simulink library "carnotUIBK_bus"  (R2023b)
settings: Solver=VariableStepAuto  StartTime=0.0  StopTime=10.0  RelTol=1e-3  EnableMultiTasking=on
values from neighbouring files (symbols this model uses):
  A = 7*10*2    (= 140)    [theta_ground_v1.m]    (also in xlswrite1.m = num2cell(data))
  amb_factor = 1    [DOOR.m]    (also in WALL.m; WINDOW.m = 0)
  area = obj.width * obj.height    [DOOR.m]    (also in RES.m = []; ROOM.m = 0; THERMALZONE.m = area + room(kk).area; WALL.m = area - obj.doors(jj).calc_area())
  B = A/(0.5 * P)    (= 8.23529411765)    [theta_ground_v1.m]
  boundary = BOUNDARY()    [BUILDING.m]    (also in WALL.m = '')
  building = obj    [BUILDING.m]    (also in create_building_automatic.m = building.save(); ini_building_automatic.m = building.add_variant_hvac(building.variant_hvac, hvac); load_building_automatic.m = building.save())
  C = zeros(1,length(d)+1)    [CONSTRUCTION.m]    (also in DOOR.m = [0 0 0]; WALL.m = [0 0 0]; WINDOW.m = [0 0 0])
  control = 2    [GAIN.m]    (also in GAINS.m)
  cp = str2num(value)    [CONSTRUCTION.m]
  height = 0    [DOOR.m]    (also in ROOM.m; THERMALZONE.m; WALL.m; WINDOW.m)
  p = [timevec_weather weather(:,12)]    [BOUNDARY.m]    (also in WEATHER.m = 0; init_carnotUIBK.m = cell2mat(carnotUIBKpaths(i,2)))
  rho = str2num(value)    [CONSTRUCTION.m]    (also in theta_ground_v1.m = 2000)
  type = 1    [CONSTRUCTION.m]    (also in GAINS.m = raw_moisture{ii,3}; STRUCTURE.m = 0)
  view_factor = 1    [DOOR.m]    (also in WINDOW.m = 0)
  wall = []    [ROOM.m]
  z = obj.Z    [WALL.m]    (also in theta_ground_v1.m = 0)
  zone = obj.zone(ind)    [THERMALZONE.m]
undefined symbols (not defined in the file or in its folder): const, Dd, get_building, mdot_air, mdot_CO2, mdot_H2O, mdot_VOC, pos, Qdot_C, Qdot_H, Qdot_I_electricity, Qdot_I_light, Qdot_I_person, Qdot_S, Qdot_T_ground, Qdot_T_internal, Qdot_T_neighbour, Qdot_T_opaque, Qdot_T_window, Qdot_V_infiltration, Qdot_V_mech, Qdot_V_window, Qdotc, Qdotr, r_frame, solar_ratio, solar_ratio1, solar_ratio2, Tc, Tr, Ts, Uvalue, wallsurface, window, window_height, window_heigth, window_width, windowsurface, x_CO2, x_H2O, x_VOC
libraries: $bdroot x134, carnot x87, simulink_extras x14, slpidlib x4, simulink x3
(part 2 of 12)

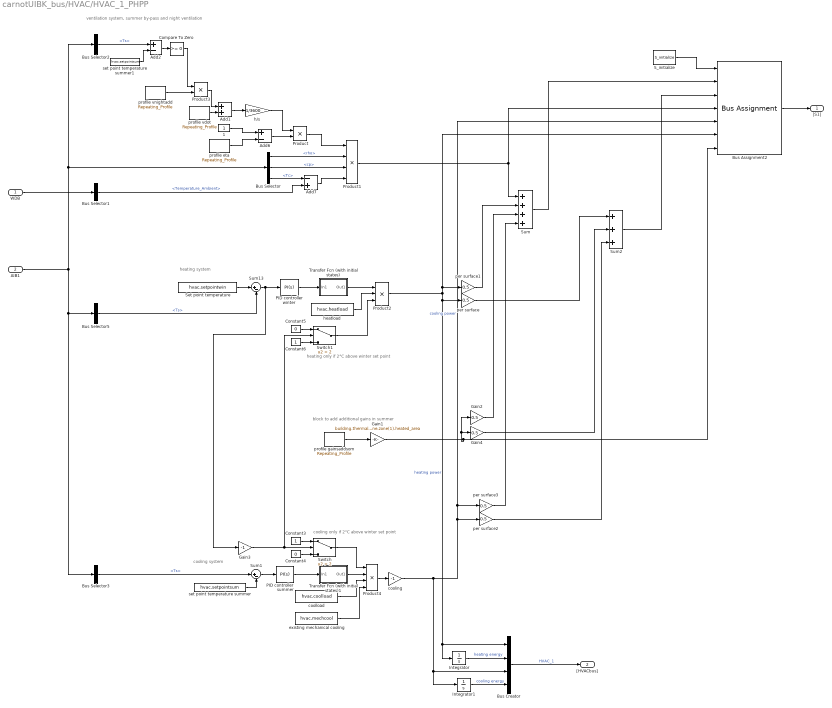
== system carnotUIBK_bus/HVAC/HVAC_1_PHPP ==
  note: cooling only if 2°C above winter set point
  note: block to add additional gains in summer
  note: heating only if 2°C above winter set point
  note: heating system
  note: cooling system
  note: ventilation system, summer by-pass and night ventilation
  WDB : Inport
  AIB1 : Inport  Port=2
  1 : Constant
  Add1 : Sum
  Add2 : Sum  Inputs=+-
  Add6 : Sum  Inputs=+-
  Add7 : Sum  Inputs=-+
  Bus Assignment2 : BusAssignment  AssignedSignals=Qdotc,Qdotr,Qdot_V_mech,Qdot_C,Qdot_H,Qdot_I_person
  Bus Creator : BusCreator  Inputs=4
  Bus Selector : BusSelector  OutputSignals=rho,cp,Tc
  Bus Selector1 : BusSelector  OutputSignals=Temperature_Ambient
  Bus Selector2 : BusSelector  OutputSignals=Ts
  Bus Selector3 : BusSelector  OutputSignals=Ts
  Bus Selector5 : BusSelector  OutputSignals=Ts
  Compare To Zero : simulink/Logic and Bit Operations/Compare To Zero  relop=>=  OutDataTypeStr=boolean
  Constant3 : Constant
  Constant4 : Constant  Value=0
  Constant5 : Constant  Value=0
  Constant6 : Constant
  Gain1 : Gain  Gain=building.thermalzone.zone(1).heated_area  SaturateOnIntegerOverflow=on  OutDataTypeStr=Inherit: Same as input  ParamDataTypeStr=Inherit: Same as input
  Gain2 : Gain  Gain=0.5  SaturateOnIntegerOverflow=on  OutDataTypeStr=Inherit: Same as input  ParamDataTypeStr=Inherit: Same as input
  Gain3 : Gain  Gain=-1  SaturateOnIntegerOverflow=on  OutDataTypeStr=Inherit: Same as input  ParamDataTypeStr=Inherit: Same as input
  Gain4 : Gain  Gain=0.5  SaturateOnIntegerOverflow=on  OutDataTypeStr=Inherit: Same as input  ParamDataTypeStr=Inherit: Same as input
  Integrator : Integrator
  Integrator1 : Integrator
  PID controller summer : slpidlib/PID Controller  Controller=PI  Form=Ideal  TimeDomain=Continuous-time  UseExternalTs=off  SampleTime=-1  IntegratorMethod=Forward Euler  FilterMethod=Forward Euler  ControllerParametersSource=internal  P=hvac.valves.Kp  I=(1/(hvac.valves.Tn*60))  UseKiTs=off  D=0  N=100  UseFilter=on  TunerSelectOption=Transfer Function Based (PID Tuner App)  InitialConditionSource=internal  InitialConditionForIntegrator=0  InitialConditionForFilter=0  DifferentiatorICPrevScaledInput=0  ExternalReset=none  TrackingMode=off  Kt=1  LimitOutput=on  SatLimitsSource=internal  UpperSaturationLimit=hvac.valves.valve_up  LowerSaturationLimit=hvac.valves.valve_low  LinearizeAsGain=off  AntiWindupMode=clamping  Kb=1  LimitIntegrator=off  UpperIntegratorSaturationLimit=inf  LowerIntegratorSaturationLimit=-inf  POutMin=[]  POutMax=[]  IOutMin=[]  IOutMax=[]  DOutMin=[]  DOutMax=[]  NOutMin=[]  NOutMax=[]  SumOutMin=[]  SumOutMax=[]  SaturationOutMin=[]  SaturationOutMax=[]  PParamMin=[]  PParamMax=[]  IParamMin=[]  IParamMax=[]  DParamMin=[]  DParamMax=[]  NParamMin=[]  NParamMax=[]  KbParamMin=[]  KbParamMax=[]  KtParamMin=[]  KtParamMax=[]  KbOutMin=[]  KbOutMax=[]  KtOutMin=[]  KtOutMax=[]  IntegratorOutMin=[]  IntegratorOutMax=[]  FilterOutMin=[]  FilterOutMax=[]  SumI1OutMin=[]  SumI1OutMax=[]  SumI2OutMin=[]  SumI2OutMax=[]  SumI3OutMin=[]  SumI3OutMax=[]  SumI4OutMin=[]  SumI4OutMax=[]  SumDOutMin=[]  SumDOutMax=[]  DifferentiatorOutMin=[]  DifferentiatorOutMax=[]  FilterDiffOutCoefMin=[]  FilterDiffOutCoefMax=[]  ReciprocalOutMin=[]  ReciprocalOutMax=[]  SumDenOutMin=[]  SumDenOutMax=[]  SumNumOutMin=[]  SumNumOutMax=[]  DivideOutMin=[]  DivideOutMax=[]  UdiffTsProdOutMin=[]  UdiffTsProdOutMax=[]  NTsProdOutMin=[]  NTsProdOutMax=[]  UintegralTsProdOutMin=[]  UintegralTsProdOutMax=[]  UngainTsProdOutMin=[]  UngainTsProdOutMax=[]  ClampingZeroOutDataTypeStr=Inherit: Inherit via back propagation  ClampingZeroOutMin=[]  ClampingZeroOutMax=[]  FilterDenConstantOutDataTypeStr=Inherit: Inherit via back propagation  FilterDenConstantOutMin=[]  FilterDenConstantOutMax=[]  PCopyOutDataTypeStr=Inherit: Inherit via back propagation  PCopyOutMin=[]  PCopyOutMax=[]  NCopyOutDataTypeStr=Inherit: Inherit via back propagation  NCopyOutMin=[]  NCopyOutMax=[]  IntegratorContinuousStateAttributes=''  IntegratorStateMustResolveToSignalObject=off  IntegratorRTWStateStorageClass=Auto  FilterContinuousStateAttributes=''  FilterStateMustResolveToSignalObject=off  FilterRTWStateStorageClass=Auto  ParallelPVariant=Passthrough  IdealPVariant=InternalParameters  IVariant=InternalParameters  DVariant=Disabled  IntegratorVariant=Continuous  SatVariant=Enabled  AWVariant=ContClampingIdeal  PCopyVariant=InternalParamsIdeal  TRVariant=Disabled  FdbkBlocksVariant=Forward  IdealPFdbkVariant=Disabled  SatFdbkVariant=Disabled  DerivativeFilterVariant=Disabled  NVariant=Disabled  NCopyVariant=Disabled_SignalSpec  FilterICVariant=Disabled  IntegratorICVariant=InternalICs  ExternalResetVariant=Disabled  TRSumVariant=Passthrough  SumFdbkVariant=Disabled  SumVariant=Sum_PI  TsampFilterVariant=InternalTs  TsampNgainVariant=Passthrough  TsampIntegralVariant=Disabled_SignalSpec  ExternalSaturationOutDataTypeStr=Inherit: Same as second input
  PID controller winter : slpidlib/PID Controller  Controller=PI  Form=Ideal  TimeDomain=Continuous-time  UseExternalTs=off  SampleTime=-1  IntegratorMethod=Forward Euler  FilterMethod=Forward Euler  ControllerParametersSource=internal  P=hvac.valves.Kp  I=(1/(hvac.valves.Tn*60))  UseKiTs=off  D=0  N=100  UseFilter=on  TunerSelectOption=Transfer Function Based (PID Tuner App)  InitialConditionSource=internal  InitialConditionForIntegrator=0  InitialConditionForFilter=0  DifferentiatorICPrevScaledInput=0  ExternalReset=none  TrackingMode=off  Kt=1  LimitOutput=on  SatLimitsSource=internal  UpperSaturationLimit=hvac.valves.valve_up  LowerSaturationLimit=hvac.valves.valve_low  LinearizeAsGain=off  AntiWindupMode=clamping  Kb=1  LimitIntegrator=off  UpperIntegratorSaturationLimit=inf  LowerIntegratorSaturationLimit=-inf  POutMin=[]  POutMax=[]  IOutMin=[]  IOutMax=[]  DOutMin=[]  DOutMax=[]  NOutMin=[]  NOutMax=[]  SumOutMin=[]  SumOutMax=[]  SaturationOutMin=[]  SaturationOutMax=[]  PParamMin=[]  PParamMax=[]  IParamMin=[]  IParamMax=[]  DParamMin=[]  DParamMax=[]  NParamMin=[]  NParamMax=[]  KbParamMin=[]  KbParamMax=[]  KtParamMin=[]  KtParamMax=[]  KbOutMin=[]  KbOutMax=[]  KtOutMin=[]  KtOutMax=[]  IntegratorOutMin=[]  IntegratorOutMax=[]  FilterOutMin=[]  FilterOutMax=[]  SumI1OutMin=[]  SumI1OutMax=[]  SumI2OutMin=[]  SumI2OutMax=[]  SumI3OutMin=[]  SumI3OutMax=[]  SumI4OutMin=[]  SumI4OutMax=[]  SumDOutMin=[]  SumDOutMax=[]  DifferentiatorOutMin=[]  DifferentiatorOutMax=[]  FilterDiffOutCoefMin=[]  FilterDiffOutCoefMax=[]  ReciprocalOutMin=[]  ReciprocalOutMax=[]  SumDenOutMin=[]  SumDenOutMax=[]  SumNumOutMin=[]  SumNumOutMax=[]  DivideOutMin=[]  DivideOutMax=[]  UdiffTsProdOutMin=[]  UdiffTsProdOutMax=[]  NTsProdOutMin=[]  NTsProdOutMax=[]  UintegralTsProdOutMin=[]  UintegralTsProdOutMax=[]  UngainTsProdOutMin=[]  UngainTsProdOutMax=[]  ClampingZeroOutDataTypeStr=Inherit: Inherit via back propagation  ClampingZeroOutMin=[]  ClampingZeroOutMax=[]  FilterDenConstantOutDataTypeStr=Inherit: Inherit via back propagation  FilterDenConstantOutMin=[]  FilterDenConstantOutMax=[]  PCopyOutDataTypeStr=Inherit: Inherit via back propagation  PCopyOutMin=[]  PCopyOutMax=[]  NCopyOutDataTypeStr=Inherit: Inherit via back propagation  NCopyOutMin=[]  NCopyOutMax=[]  IntegratorContinuousStateAttributes=''  IntegratorStateMustResolveToSignalObject=off  IntegratorRTWStateStorageClass=Auto  FilterContinuousStateAttributes=''  FilterStateMustResolveToSignalObject=off  FilterRTWStateStorageClass=Auto  ParallelPVariant=Passthrough  IdealPVariant=InternalParameters  IVariant=InternalParameters  DVariant=Disabled  IntegratorVariant=Continuous  SatVariant=Enabled  AWVariant=ContClampingIdeal  PCopyVariant=InternalParamsIdeal  TRVariant=Disabled  FdbkBlocksVariant=Forward  IdealPFdbkVariant=Disabled  SatFdbkVariant=Disabled  DerivativeFilterVariant=Disabled  NVariant=Disabled  NCopyVariant=Disabled_SignalSpec  FilterICVariant=Disabled  IntegratorICVariant=InternalICs  ExternalResetVariant=Disabled  TRSumVariant=Passthrough  SumFdbkVariant=Disabled  SumVariant=Sum_PI  TsampFilterVariant=InternalTs  TsampNgainVariant=Passthrough  TsampIntegralVariant=Disabled_SignalSpec  ExternalSaturationOutDataTypeStr=Inherit: Same as second input
  Product : Product
  Product1 : Product  Inputs=4
  Product2 : Product  Inputs=3
  Product3 : Product
  Product4 : Product  Inputs=4
  S_initialize : $bdroot/general/S_initialize  SystemSampleTime=-1  VariantActivationTime=update diagram  AllowFlexibleInterface=on  Latency=0  AutoFrameSizeCalculation=off
  Set point temperature : Constant  Value=hvac.setpointwin  VectorParams1D=off
  Sum : Sum  Inputs=++++
  Sum1 : Sum  Inputs=|+-
  Sum13 : Sum  Inputs=|+-
  Sum2 : Sum  Inputs=+++
  Switch : Switch  Criteria=u2 > Threshold  Threshold=2  SaturateOnIntegerOverflow=off  InputSameDT=off
  Switch1 : Switch  Criteria=u2 > Threshold  Threshold=2  SaturateOnIntegerOverflow=off  InputSameDT=off
  Transfer Fcn (with initial states) : Subsystem  mask(Transfer Function with Initial States){N=[1], D=[300  1], X0=0}
      mask prompts: N "Numerator:"; D "Denominator:"; X0 "Initial conditions:"
      mask help: Vector expressions for numerator, and denominator. Coefficients are in descending powers of s.
      mask init:
      | [A,B,C,Dd]=tf2ss(N,D);if (isempty(X0));[m,n]=size(A);X0=zeros(1,m); end;
      mask Help: Specify the initial states for the transfer function.  The state ordering is determined by the m-file tf2ss.  There is no unique mapping of the states in a transfer function to states in a state-space representation.  However, tf2ss will consistently use the same mapping for a given transfer function.
      mask Display: dpoly(N,D,'s')
  Transfer Fcn (with initial states)1 : Subsystem  mask(Transfer Function with Initial States){N=[1], D=[300  1], X0=0}
      mask prompts: N "Numerator:"; D "Denominator:"; X0 "Initial conditions:"
      mask help: Vector expressions for numerator, and denominator. Coefficients are in descending powers of s.
      mask init:
      | [A,B,C,Dd]=tf2ss(N,D);if (isempty(X0));[m,n]=size(A);X0=zeros(1,m); end;
      mask Help: Specify the initial states for the transfer function.  The state ordering is determined by the m-file tf2ss.  There is no unique mapping of the states in a transfer function to states in a state-space representation.  However, tf2ss will consistently use the same mapping for a given transfer function.
      mask Display: dpoly(N,D,'s')
  cooling : Gain  Gain=-1  SaturateOnIntegerOverflow=on  OutDataTypeStr=Inherit: Same as input  ParamDataTypeStr=Inherit: Same as input
  coolload : Constant  Value=hvac.coolload
  existing mechanical cooling : Constant  Value=hvac.mechcool
  h/s : Gain  Gain=1/3600
  heatload : Constant  Value=hvac.heatload
  per surface{,1..3} (4 alike) : Gain  Gain=0.5  SaturateOnIntegerOverflow=on  OutDataTypeStr=Inherit: Same as input  ParamDataTypeStr=Inherit: Same as input
  profile eta : carnot/Load/General/Repeating_Profile  period=hvac.eta.time(end)  rep_seq_t=hvac.eta.time(1:end-1)  rep_seq_d=hvac.eta.duration  rep_seq_y=hvac.eta.value
      settings: SourceProductName=Carnot
  profile gainsaddsom : carnot/Load/General/Repeating_Profile  period=hvac.gainsum.time(end)  rep_seq_t=hvac.gainsum.time(1:end-1)  rep_seq_d=hvac.gainsum.duration  rep_seq_y=hvac.gainsum.value
      settings: SourceProductName=Carnot
  profile vdot : carnot/Load/General/Repeating_Profile  period=hvac.vdot_winsom.time(end)  rep_seq_t=hvac.vdot_winsom.time(1:end-1)  rep_seq_d=hvac.vdot_winsom.duration  rep_seq_y=hvac.vdot_winsom.value
      settings: SourceProductName=Carnot
  profile vnightadd : carnot/Load/General/Repeating_Profile  period=hvac.night_vent_s.time(end)  rep_seq_t=hvac.night_vent_s.time(1:end-1)  rep_seq_d=hvac.night_vent_s.duration  rep_seq_y=hvac.night_vent_s.value
      settings: SourceProductName=Carnot
  set point temperature summer : Constant  Value=hvac.setpointsum  VectorParams1D=off
  set point temperature summer1 : Constant  Value=hvac.setpointsum  VectorParams1D=off
  "[S1]" : Outport  InitialOutput=0  VectorParamsAs1DForOutWhenUnconnected=off
  "[HVACbus]" : Outport  Port=2  InitialOutput=0  VectorParamsAs1DForOutWhenUnconnected=off
  wires:
  profile eta/1 -> Add6/2
  profile vdot/1 -> Add1/2
  1/1 -> Add6/1
  Add6/1 -> Product/2
  Product/1 -> Product1/1
  Bus Selector/1 -> Product1/2  "<rho>"
  Bus Selector/2 -> Product1/3  "<cp>"
  Bus Selector/3 -> Add7/1  "<Tc>"
  Product1/1 -> Sum/1, Bus Assignment2/4
  WDB/1 -> Bus Selector1/1
  Bus Selector1/1 -> Add7/2  "<Temperature_Ambient>"
  Add7/1 -> Product1/4
  h/s/1 -> Product/1
  Sum13/1 -> PID controller winter/1, Gain3/1
  Set point temperature/1 -> Sum13/1
  Bus Selector5/1 -> Sum13/2  "<Ts>"
  PID controller winter/1 -> Transfer Fcn (with initial states)/1(In1)
  heatload/1 -> Product2/2
  per surface/1 -> Sum2/1
  per surface1/1 -> Sum/2
  Transfer Fcn (with initial states)/1(Out1) -> Product2/1
  Add1/1 -> h/s/1
  Product3/1 -> Add1/1
  profile vnightadd/1 -> Product3/2
  Bus Selector2/1 -> Add2/1  "<Ts>"
  set point temperature summer1/1 -> Add2/2
  Add2/1 -> Compare To Zero/1
  Compare To Zero/1 -> Product3/1
  profile gainsaddsom/1 -> Gain1/1
  Gain1/1 -> Gain2/1, Gain4/1, Bus Assignment2/7
  Sum1/1 -> PID controller summer/1
  set point temperature summer/1 -> Sum1/2
  Bus Selector3/1 -> Sum1/1  "<Ts>"
  PID controller summer/1 -> Transfer Fcn (with initial states)1/1(In1)
  coolload/1 -> Product4/3
  Product4/1 -> cooling/1
  per surface2/1 -> Sum2/3
  per surface3/1 -> Sum/4
  Transfer Fcn (with initial states)1/1(Out1) -> Product4/2
  AIB1/1 -> Bus Selector3/1, Bus Selector5/1, Bus Selector/1, Bus Selector2/1
  existing mechanical cooling/1 -> Product4/4
  Constant3/1 -> Switch/1
  Constant4/1 -> Switch/3
  Switch/1 -> Product4/1
  Gain3/1 -> Switch1/2, Switch/2
  Constant5/1 -> Switch1/1
  Constant6/1 -> Switch1/3
  Switch1/1 -> Product2/3
  Bus Creator/1 -> "[HVACbus]"/1  "HVAC_1"
  Integrator/1 -> Bus Creator/2  "heating energy"
  Product2/1 -> Bus Assignment2/6, per surface1/1, Integrator/1, Bus Creator/1, per surface/1  "heating power"
  Integrator1/1 -> Bus Creator/4  "cooling energy"
  cooling/1 -> Bus Creator/3, Integrator1/1, Bus Assignment2/5, per surface3/1, per surface2/1  "cooling power"
  S_initialize/1 -> Bus Assignment2/1
  Gain2/1 -> Sum/3
  Gain4/1 -> Sum2/2
  Sum/1 -> Bus Assignment2/2
  Sum2/1 -> Bus Assignment2/3
  Bus Assignment2/1 -> "[S1]"/1

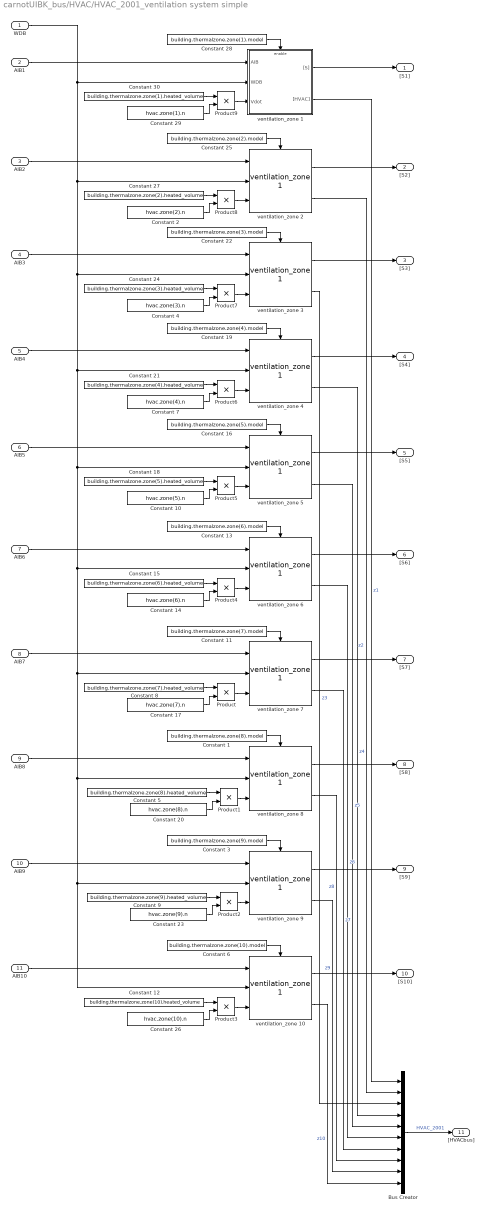
== system carnotUIBK_bus/HVAC/HVAC_2001_ventilation system simple ==
  WDB : Inport
  AIB1 : Inport  Port=2
  AIB2 : Inport  Port=3
  AIB3 : Inport  Port=4
  AIB4 : Inport  Port=5
  AIB5 : Inport  Port=6
  AIB6 : Inport  Port=7
  AIB7 : Inport  Port=8
  "AIB8 " : Inport  Port=9
  AIB9 : Inport  Port=10
  AIB10 : Inport  Port=11
  Bus Creator : BusCreator  Inputs=10
  Constant 1 : Constant  Value=building.thermalzone.zone(8).model  VectorParams1D=off
  Constant 10 : Constant  Value=hvac.zone(5).n  VectorParams1D=off
  Constant 11 : Constant  Value=building.thermalzone.zone(7).model  VectorParams1D=off
  Constant 12 : Constant  Value=building.thermalzone.zone(10).heated_volume  VectorParams1D=off
  Constant 13 : Constant  Value=building.thermalzone.zone(6).model  VectorParams1D=off
  Constant 14 : Constant  Value=hvac.zone(6).n  VectorParams1D=off
  Constant 15 : Constant  Value=building.thermalzone.zone(6).heated_volume  VectorParams1D=off
  Constant 16 : Constant  Value=building.thermalzone.zone(5).model  VectorParams1D=off
  Constant 17 : Constant  Value=hvac.zone(7).n  VectorParams1D=off
  Constant 18 : Constant  Value=building.thermalzone.zone(5).heated_volume  VectorParams1D=off
  Constant 19 : Constant  Value=building.thermalzone.zone(4).model  VectorParams1D=off
  Constant 2 : Constant  Value=hvac.zone(2).n  VectorParams1D=off
  Constant 20 : Constant  Value=hvac.zone(8).n  VectorParams1D=off
  Constant 21 : Constant  Value=building.thermalzone.zone(4).heated_volume  VectorParams1D=off
  Constant 22 : Constant  Value=building.thermalzone.zone(3).model  VectorParams1D=off
  Constant 23 : Constant  Value=hvac.zone(9).n  VectorParams1D=off
  Constant 24 : Constant  Value=building.thermalzone.zone(3).heated_volume  VectorParams1D=off
  Constant 25 : Constant  Value=building.thermalzone.zone(2).model  VectorParams1D=off
  Constant 26 : Constant  Value=hvac.zone(10).n  VectorParams1D=off
  Constant 27 : Constant  Value=building.thermalzone.zone(2).heated_volume  VectorParams1D=off
  Constant 28 : Constant  Value=building.thermalzone.zone(1).model  VectorParams1D=off
  Constant 29 : Constant  Value=hvac.zone(1).n  VectorParams1D=off
  Constant 3 : Constant  Value=building.thermalzone.zone(9).model  VectorParams1D=off
  Constant 30 : Constant  Value=building.thermalzone.zone(1).heated_volume  VectorParams1D=off
  Constant 4 : Constant  Value=hvac.zone(3).n  VectorParams1D=off
  Constant 5 : Constant  Value=building.thermalzone.zone(8).heated_volume  VectorParams1D=off
  Constant 6 : Constant  Value=building.thermalzone.zone(10).model  VectorParams1D=off
  Constant 7 : Constant  Value=hvac.zone(4).n  VectorParams1D=off
  Constant 8 : Constant  Value=building.thermalzone.zone(7).heated_volume  VectorParams1D=off
  Constant 9 : Constant  Value=building.thermalzone.zone(9).heated_volume  VectorParams1D=off
  Product{,1..9} (10 alike) : Product
  ventilation_zone 1 : Subsystem  mask(ACTIVE COMPONENT){co2=400, eta=hvac.zone(1).eta, eta_x=hvac.zone(1).eta_x}
      mask prompts: co2 "CO2 content of air in ppm"; eta "heat recovery efficiency"; eta_x "moisture recovery efficiency"
      mask help:
      | This block represents the AIR VENTILATION from outdoors into a zone.
      |
      | r : rate of nominal air flow between outdoors and indoor, [0,1]
      | [S] : vector for sinks and sources.
      |
      | NOTE: Mass flows of water and CO2 are taken into consideration.
      |
      | ASSUMPTION:
      | Incoming air volume flow is identical to outgoing air volume flow.
      mask init:
      | CO2norm = co2*1e-6;
      mask Help: web(fullfile(path_carnot('help'),'Ventilation_AIV.html'),'-helpbrowser')
      mask Display:
      | plot([0.2 0.35], [0.8 0.7])
      | plot([0.35 0.65], [0.7 0.7])
      | plot([0.65 0.8], [0.7 0.8])
      | plot([0.65 0.8], [0.76 0.8])
      | plot([0.7 0.8], [0.65 0.8])
      | 
      | plot([0.2 0.35], [0.2 0.3])
      | plot([0.35 0.65], [0.3 0.3])
      | plot([0.65 0.8], [0.3 0.2])
      | plot([0.2 0.25], [0.2 0.32])
      | plot([0.2 0.35], [0.2 0.23])
      | 
      | plot ([0.45 0.45], [0 1])
      | plot ([0.55 0.55], [0 1])
      | 
      | plot ([0.45 0.55], [0.2 0.2])
      | plot ([0.45 0.55], [0.8 0.8])
      | 
      | plot ([0.45 0.55], [0 0.2])
      | plot ([0.45 0.55], [0.8 1])
  ventilation_zone 10 : $bdroot/HVAC/HVAC_2001_ventilation system simple/ventilation_zone 1  co2=400  eta=hvac.zone(10).eta  eta_x=hvac.zone(10).eta_x
  ventilation_zone 2 : $bdroot/HVAC/HVAC_2001_ventilation system simple/ventilation_zone 1  co2=400  eta=hvac.zone(2).eta  eta_x=hvac.zone(2).eta_x
  ventilation_zone 3 : $bdroot/HVAC/HVAC_2001_ventilation system simple/ventilation_zone 1  co2=400  eta=hvac.zone(3).eta  eta_x=hvac.zone(3).eta_x
  ventilation_zone 4 : $bdroot/HVAC/HVAC_2001_ventilation system simple/ventilation_zone 1  co2=400  eta=hvac.zone(4).eta  eta_x=hvac.zone(4).eta_x
  ventilation_zone 5 : $bdroot/HVAC/HVAC_2001_ventilation system simple/ventilation_zone 1  co2=400  eta=hvac.zone(5).eta  eta_x=hvac.zone(5).eta_x
  ventilation_zone 6 : $bdroot/HVAC/HVAC_2001_ventilation system simple/ventilation_zone 1  co2=400  eta=hvac.zone(6).eta  eta_x=hvac.zone(6).eta_x
  ventilation_zone 7 : $bdroot/HVAC/HVAC_2001_ventilation system simple/ventilation_zone 1  co2=400  eta=hvac.zone(7).eta  eta_x=hvac.zone(7).eta_x
  ventilation_zone 8 : $bdroot/HVAC/HVAC_2001_ventilation system simple/ventilation_zone 1  co2=400  eta=hvac.zone(8).eta  eta_x=hvac.zone(8).eta_x
  ventilation_zone 9 : $bdroot/HVAC/HVAC_2001_ventilation system simple/ventilation_zone 1  co2=400  eta=hvac.zone(9).eta  eta_x=hvac.zone(9).eta_x
  "[S1]" : Outport  VectorParamsAs1DForOutWhenUnconnected=off
  "[S2]" : Outport  Port=2  VectorParamsAs1DForOutWhenUnconnected=off
  "[S3]" : Outport  Port=3  VectorParamsAs1DForOutWhenUnconnected=off
  "[S4]" : Outport  Port=4  VectorParamsAs1DForOutWhenUnconnected=off
  "[S5]" : Outport  Port=5  VectorParamsAs1DForOutWhenUnconnected=off
  "[S6]" : Outport  Port=6  VectorParamsAs1DForOutWhenUnconnected=off
  "[S7]" : Outport  Port=7  VectorParamsAs1DForOutWhenUnconnected=off
  "[S8]" : Outport  Port=8  VectorParamsAs1DForOutWhenUnconnected=off
  "[S9]" : Outport  Port=9  VectorParamsAs1DForOutWhenUnconnected=off
  "[S10]" : Outport  Port=10  VectorParamsAs1DForOutWhenUnconnected=off
  "[HVACbus]" : Outport  Port=11  InitialOutput=0  VectorParamsAs1DForOutWhenUnconnected=off
  wires:
  AIB7/1 -> ventilation_zone 7/1
  ventilation_zone 7/1 -> "[S7]"/1
  Constant 11/1 -> ventilation_zone 7/Enable
  "AIB8 "/1 -> ventilation_zone 8/1
  Product1/1 -> ventilation_zone 8/3
  ventilation_zone 8/1 -> "[S8]"/1
  Constant 1/1 -> ventilation_zone 8/Enable
  AIB9/1 -> ventilation_zone 9/1
  Product2/1 -> ventilation_zone 9/3
  ventilation_zone 9/1 -> "[S9]"/1
  Constant 3/1 -> ventilation_zone 9/Enable
  AIB10/1 -> ventilation_zone 10/1
  Product3/1 -> ventilation_zone 10/3
  ventilation_zone 10/1 -> "[S10]"/1
  Constant 6/1 -> ventilation_zone 10/Enable
  Constant 8/1 -> Product/1
  Product/1 -> ventilation_zone 7/3
  Constant 17/1 -> Product/2
  Constant 5/1 -> Product1/1
  Constant 20/1 -> Product1/2
  Constant 9/1 -> Product2/1
  Constant 23/1 -> Product2/2
  Constant 12/1 -> Product3/1
  Constant 26/1 -> Product3/2
  AIB6/1 -> ventilation_zone 6/1
  ventilation_zone 6/1 -> "[S6]"/1
  Constant 13/1 -> ventilation_zone 6/Enable
  Constant 15/1 -> Product4/1
  Product4/1 -> ventilation_zone 6/3
  Constant 14/1 -> Product4/2
  AIB5/1 -> ventilation_zone 5/1
  ventilation_zone 5/1 -> "[S5]"/1
  Constant 16/1 -> ventilation_zone 5/Enable
  Constant 18/1 -> Product5/1
  Product5/1 -> ventilation_zone 5/3
  Constant 10/1 -> Product5/2
  AIB4/1 -> ventilation_zone 4/1
  ventilation_zone 4/1 -> "[S4]"/1
  Constant 19/1 -> ventilation_zone 4/Enable
  Constant 21/1 -> Product6/1
  Product6/1 -> ventilation_zone 4/3
  Constant 7/1 -> Product6/2
  AIB3/1 -> ventilation_zone 3/1
  ventilation_zone 3/1 -> "[S3]"/1
  Constant 22/1 -> ventilation_zone 3/Enable
  Constant 24/1 -> Product7/1
  Product7/1 -> ventilation_zone 3/3
  Constant 4/1 -> Product7/2
  AIB2/1 -> ventilation_zone 2/1
  ventilation_zone 2/1 -> "[S2]"/1
  Constant 25/1 -> ventilation_zone 2/Enable
  Constant 27/1 -> Product8/1
  Product8/1 -> ventilation_zone 2/3
  Constant 2/1 -> Product8/2
  AIB1/1 -> ventilation_zone 1/1(AIB)
  ventilation_zone 1/1("[S]") -> "[S1]"/1
  Constant 28/1 -> ventilation_zone 1/Enable
  WDB/1 -> ventilation_zone 1/2(WDB), ventilation_zone 2/2, ventilation_zone 3/2, ventilation_zone 4/2, ventilation_zone 5/2, ventilation_zone 6/2, ventilation_zone 7/2, ventilation_zone 8/2, ventilation_zone 10/2, ventilation_zone 9/2
  Constant 30/1 -> Product9/1
  Product9/1 -> ventilation_zone 1/3(Vdot)
  Constant 29/1 -> Product9/2
  Bus Creator/1 -> "[HVACbus]"/1  "HVAC_2001"
  ventilation_zone 1/2("[HVAC]") -> Bus Creator/1  "z1"
  ventilation_zone 2/2 -> Bus Creator/2  "z2"
  ventilation_zone 3/2 -> Bus Creator/3  "z3"
  ventilation_zone 4/2 -> Bus Creator/4  "z4"
  ventilation_zone 5/2 -> Bus Creator/5  "z5"
  ventilation_zone 6/2 -> Bus Creator/6  "z6"
  ventilation_zone 7/2 -> Bus Creator/7  "z7"
  ventilation_zone 8/2 -> Bus Creator/8  "z8"
  ventilation_zone 9/2 -> Bus Creator/9  "z9"
  ventilation_zone 10/2 -> Bus Creator/10  "z10"

== system carnotUIBK_bus/HVAC/HVAC_9001_window shading ==
  WDB : Inport
  Bus Selector : BusSelector  OutputSignals=Solar_Radiation_beam_normal
  Switch : Switch  Criteria=u2 > Threshold  Threshold=hvac.window(1).I_glob  SaturateOnIntegerOverflow=off  InputSameDT=off
  Switch1 : Switch  Criteria=u2 > Threshold  Threshold=hvac.window(2).I_glob  SaturateOnIntegerOverflow=off  InputSameDT=off
  Switch2 : Switch  Criteria=u2 > Threshold  Threshold=hvac.window(3).I_glob  SaturateOnIntegerOverflow=off  InputSameDT=off
  Switch3 : Switch  Criteria=u2 > Threshold  Threshold=hvac.window(4).I_glob  SaturateOnIntegerOverflow=off  InputSameDT=off
  Switch4 : Switch  Criteria=u2 > Threshold  Threshold=hvac.window(5).I_glob  SaturateOnIntegerOverflow=off  InputSameDT=off
  Switch5 : Switch  Criteria=u2 > Threshold  Threshold=hvac.window(6).I_glob  SaturateOnIntegerOverflow=off  InputSameDT=off
  Transfer Fcn (with initial states) : Subsystem  mask(Transfer Function with Initial States){N=[1], D=[600 1], X0=0}
      mask prompts: N "Numerator:"; D "Denominator:"; X0 "Initial conditions:"
      mask help: Vector expressions for numerator, and denominator. Coefficients are in descending powers of s.
      mask init:
      | [A,B,C,Dd]=tf2ss(N,D);if (isempty(X0));[m,n]=size(A);X0=zeros(1,m); end;
      mask Help: Specify the initial states for the transfer function.  The state ordering is determined by the m-file tf2ss.  There is no unique mapping of the states in a transfer function to states in a state-space representation.  However, tf2ss will consistently use the same mapping for a given transfer function.
      mask Display: dpoly(N,D,'s')
  Window shading zone 1 : carnot/Load/General/Repeating_Profile  period=hvac.window(1).timevalues(end)  rep_seq_t=hvac.window(1).timevalues(1:end-1)  rep_seq_d=hvac.window(1).timeduration  rep_seq_y=hvac.window(1).values
      settings: SourceProductName=Carnot
  Window shading zone 2 : carnot/Load/General/Repeating_Profile  period=hvac.window(2).timevalues(end)  rep_seq_t=hvac.window(2).timevalues(1:end-1)  rep_seq_d=hvac.window(2).timeduration  rep_seq_y=hvac.window(2).values
      settings: SourceProductName=Carnot
  Window shading zone 3 : carnot/Load/General/Repeating_Profile  period=hvac.window(3).timevalues(end)  rep_seq_t=hvac.window(3).timevalues(1:end-1)  rep_seq_d=hvac.window(3).timeduration  rep_seq_y=hvac.window(3).values
      settings: SourceProductName=Carnot
  Window shading zone 4 : carnot/Load/General/Repeating_Profile  period=hvac.window(4).timevalues(end)  rep_seq_t=hvac.window(4).timevalues(1:end-1)  rep_seq_d=hvac.window(4).timeduration  rep_seq_y=hvac.window(4).values
      settings: SourceProductName=Carnot
  Window shading zone 5 : carnot/Load/General/Repeating_Profile  period=hvac.window(5).timevalues(end)  rep_seq_t=hvac.window(5).timevalues(1:end-1)  rep_seq_d=hvac.window(5).timeduration  rep_seq_y=hvac.window(5).values
      settings: SourceProductName=Carnot
  Window shading zone 6 : carnot/Load/General/Repeating_Profile  period=hvac.window(6).timevalues(end)  rep_seq_t=hvac.window(6).timevalues(1:end-1)  rep_seq_d=hvac.window(6).timeduration  rep_seq_y=hvac.window(6).values
      settings: SourceProductName=Carnot
  no shading : Constant  Value=0
  ctrl 1 : Outport  VectorParamsAs1DForOutWhenUnconnected=off
  ctrl 2 : Outport  Port=2  VectorParamsAs1DForOutWhenUnconnected=off
  ctrl 3 : Outport  Port=3  VectorParamsAs1DForOutWhenUnconnected=off
  ctrl 4 : Outport  Port=4  VectorParamsAs1DForOutWhenUnconnected=off
  ctrl 5 : Outport  Port=5  VectorParamsAs1DForOutWhenUnconnected=off
  ctrl 6 : Outport  Port=6  VectorParamsAs1DForOutWhenUnconnected=off
  wires:
  WDB/1 -> Bus Selector/1
  Switch/1 -> ctrl 1/1
  Window shading zone 1/1 -> Switch/1
  Bus Selector/1 -> Transfer Fcn (with initial states)/1(In1)  "<Solar_Radiation_beam_normal>"
  Switch3/1 -> ctrl 4/1
  Window shading zone 4/1 -> Switch3/1
  Switch1/1 -> ctrl 2/1
  Window shading zone 2/1 -> Switch1/1
  Switch4/1 -> ctrl 5/1
  Window shading zone 5/1 -> Switch4/1
  Switch5/1 -> ctrl 6/1
  Window shading zone 6/1 -> Switch5/1
  no shading/1 -> Switch5/3, Switch4/3, Switch3/3, Switch2/3, Switch/3, Switch1/3
  Switch2/1 -> ctrl 3/1
  Window shading zone 3/1 -> Switch2/1
  Transfer Fcn (with initial states)/1(Out1) -> Switch2/2, Switch3/2, Switch5/2, Switch4/2, Switch1/2, Switch/2

== system carnotUIBK_bus/HVAC/HVAC_9002_window opening ==
  WDB : Inport
  AIB window 1 : Inport  Port=2
  AIB window 2 : Inport  Port=3
  AIB window 3 : Inport  Port=4
  AIB window 4 : Inport  Port=5
  AIB window 5 : Inport  Port=6
  AIB window 6 : Inport  Port=7
  Constant 1 : Constant  Value=hvac.window(2).setpoint  VectorParams1D=off
  Constant 2 : Constant  Value=hvac.window(3).setpoint  VectorParams1D=off
  Constant 3 : Constant  Value=hvac.window(4).setpoint  VectorParams1D=off
  Constant 4 : Constant  Value=hvac.window(5).setpoint  VectorParams1D=off
  Constant 5 : Constant  Value=hvac.window(6).setpoint  VectorParams1D=off
  Constant 6 : Constant  Value=hvac.window(1).setpoint  VectorParams1D=off
  on{,1..5} (6 alike) : Constant
  window opening 1 : Subsystem
  window opening 2 : Subsystem
  window opening 3 : Subsystem
  window opening 4 : Subsystem
  window opening 5 : Subsystem
  window opening 6 : Subsystem
  ctrl 1 : Outport  VectorParamsAs1DForOutWhenUnconnected=off
  ctrl 2 : Outport  Port=2  VectorParamsAs1DForOutWhenUnconnected=off
  ctrl 3 : Outport  Port=3  VectorParamsAs1DForOutWhenUnconnected=off
  ctrl 4 : Outport  Port=4  VectorParamsAs1DForOutWhenUnconnected=off
  ctrl 5 : Outport  Port=5  VectorParamsAs1DForOutWhenUnconnected=off
  ctrl 6 : Outport  Port=6  VectorParamsAs1DForOutWhenUnconnected=off
  wires:
  AIB window 1/1 -> window opening 1/2(AIB)
  window opening 1/1(state) -> ctrl 1/1
  on2/1 -> window opening 1/Enable
  AIB window 2/1 -> window opening 2/2(AIB)
  window opening 2/1(state) -> ctrl 2/1
  on1/1 -> window opening 2/Enable
  AIB window 4/1 -> window opening 4/2(AIB)
  window opening 4/1(state) -> ctrl 4/1
  on/1 -> window opening 4/Enable
  AIB window 5/1 -> window opening 5/2(AIB)
  window opening 5/1(state) -> ctrl 5/1
  on3/1 -> window opening 5/Enable
  Constant 6/1 -> window opening 1/1(setpoint)
  AIB window 6/1 -> window opening 6/2(AIB)
  window opening 6/1(state) -> ctrl 6/1
  on4/1 -> window opening 6/Enable
  Constant 1/1 -> window opening 2/1(setpoint)
  Constant 3/1 -> window opening 4/1(setpoint)
  Constant 4/1 -> window opening 5/1(setpoint)
  Constant 5/1 -> window opening 6/1(setpoint)
  WDB/1 -> window opening 6/3(WDB), window opening 5/3(WDB), window opening 4/3(WDB), window opening 3/3(WDB), window opening 2/3(WDB), window opening 1/3(WDB)
  AIB window 3/1 -> window opening 3/2(AIB)
  window opening 3/1(state) -> ctrl 3/1
  on5/1 -> window opening 3/Enable
  Constant 2/1 -> window opening 3/1(setpoint)

== system carnotUIBK_bus/HVAC/HVAC_9003_door opening ==
  profile opening door 1 : carnot/Load/General/Repeating_Profile  period=hvac.door(1).timevalues(end)  rep_seq_t=hvac.door(1).timevalues(1:end-1)  rep_seq_d=hvac.door(1).timeduration  rep_seq_y=hvac.door(1).values
      settings: SourceProductName=Carnot
  profile opening door 2 : carnot/Load/General/Repeating_Profile  period=hvac.door(2).timevalues(end)  rep_seq_t=hvac.door(2).timevalues(1:end-1)  rep_seq_d=hvac.door(2).timeduration  rep_seq_y=hvac.door(2).values
      settings: SourceProductName=Carnot
  profile opening door 3 : carnot/Load/General/Repeating_Profile  period=hvac.door(3).timevalues(end)  rep_seq_t=hvac.door(3).timevalues(1:end-1)  rep_seq_d=hvac.door(3).timeduration  rep_seq_y=hvac.door(3).values
      settings: SourceProductName=Carnot
  profile opening door 4 : carnot/Load/General/Repeating_Profile  period=hvac.door(4).timevalues(end)  rep_seq_t=hvac.door(4).timevalues(1:end-1)  rep_seq_d=hvac.door(4).timeduration  rep_seq_y=hvac.door(4).values
      settings: SourceProductName=Carnot
  profile opening door 5 : carnot/Load/General/Repeating_Profile  period=hvac.door(5).timevalues(end)  rep_seq_t=hvac.door(5).timevalues(1:end-1)  rep_seq_d=hvac.door(5).timeduration  rep_seq_y=hvac.door(5).values
      settings: SourceProductName=Carnot
  profile opening door 6 : carnot/Load/General/Repeating_Profile  period=hvac.door(6).timevalues(end)  rep_seq_t=hvac.door(6).timevalues(1:end-1)  rep_seq_d=hvac.door(6).timeduration  rep_seq_y=hvac.door(6).values
      settings: SourceProductName=Carnot
  ctrl 1 : Outport  VectorParamsAs1DForOutWhenUnconnected=off
  ctrl 2 : Outport  Port=2  VectorParamsAs1DForOutWhenUnconnected=off
  ctrl 3 : Outport  Port=3  VectorParamsAs1DForOutWhenUnconnected=off
  ctrl 4 : Outport  Port=4  VectorParamsAs1DForOutWhenUnconnected=off
  ctrl 5 : Outport  Port=5  VectorParamsAs1DForOutWhenUnconnected=off
  ctrl 6 : Outport  Port=6  VectorParamsAs1DForOutWhenUnconnected=off
  wires:
  profile opening door 1/1 -> ctrl 1/1
  profile opening door 2/1 -> ctrl 2/1
  profile opening door 4/1 -> ctrl 4/1
  profile opening door 5/1 -> ctrl 5/1
  profile opening door 6/1 -> ctrl 6/1
  profile opening door 3/1 -> ctrl 3/1

== system carnotUIBK_bus/HVAC/HVAC_999_TEMPLATE ==
  note: PLEASE CHANGE THE THIS TO THE SYSTEM NUMBER!
  WDB : Inport
  AIB1 : Inport  Port=2
  AIB2 : Inport  Port=3
  Bus Assignment2 : BusAssignment  AssignedSignals=Qdotc,Qdotr,Qdot_H
  Bus Creator : BusCreator  Inputs=2
  Bus Selector1 : BusSelector  OutputSignals=Temperature_Ambient
  Bus Selector3 : BusSelector  OutputSignals=Ts
  Integrator : Integrator
  PID controller : slpidlib/PID Controller  Controller=PI  Form=Ideal  TimeDomain=Continuous-time  UseExternalTs=off  SampleTime=-1  IntegratorMethod=Forward Euler  FilterMethod=Forward Euler  ControllerParametersSource=internal  P=hvac.PID.Kp  I=(1/(hvac.PID.Tn*60))  UseKiTs=off  D=0  N=100  UseFilter=on  TunerSelectOption=Transfer Function Based (PID Tuner App)  InitialConditionSource=internal  InitialConditionForIntegrator=0  InitialConditionForFilter=0  DifferentiatorICPrevScaledInput=0  ExternalReset=none  TrackingMode=off  Kt=1  LimitOutput=on  SatLimitsSource=internal  UpperSaturationLimit=hvac.valves.valve_up  LowerSaturationLimit=hvac.valves.valve_low  LinearizeAsGain=off  AntiWindupMode=clamping  Kb=1  LimitIntegrator=off  UpperIntegratorSaturationLimit=inf  LowerIntegratorSaturationLimit=-inf  POutMin=[]  POutMax=[]  IOutMin=[]  IOutMax=[]  DOutMin=[]  DOutMax=[]  NOutMin=[]  NOutMax=[]  SumOutMin=[]  SumOutMax=[]  SaturationOutMin=[]  SaturationOutMax=[]  PParamMin=[]  PParamMax=[]  IParamMin=[]  IParamMax=[]  DParamMin=[]  DParamMax=[]  NParamMin=[]  NParamMax=[]  KbParamMin=[]  KbParamMax=[]  KtParamMin=[]  KtParamMax=[]  KbOutMin=[]  KbOutMax=[]  KtOutMin=[]  KtOutMax=[]  IntegratorOutMin=[]  IntegratorOutMax=[]  FilterOutMin=[]  FilterOutMax=[]  SumI1OutMin=[]  SumI1OutMax=[]  SumI2OutMin=[]  SumI2OutMax=[]  SumI3OutMin=[]  SumI3OutMax=[]  SumI4OutMin=[]  SumI4OutMax=[]  SumDOutMin=[]  SumDOutMax=[]  DifferentiatorOutMin=[]  DifferentiatorOutMax=[]  FilterDiffOutCoefMin=[]  FilterDiffOutCoefMax=[]  ReciprocalOutMin=[]  ReciprocalOutMax=[]  SumDenOutMin=[]  SumDenOutMax=[]  SumNumOutMin=[]  SumNumOutMax=[]  DivideOutMin=[]  DivideOutMax=[]  UdiffTsProdOutMin=[]  UdiffTsProdOutMax=[]  NTsProdOutMin=[]  NTsProdOutMax=[]  UintegralTsProdOutMin=[]  UintegralTsProdOutMax=[]  UngainTsProdOutMin=[]  UngainTsProdOutMax=[]  ClampingZeroOutDataTypeStr=Inherit: Inherit via back propagation  ClampingZeroOutMin=[]  ClampingZeroOutMax=[]  FilterDenConstantOutDataTypeStr=Inherit: Inherit via back propagation  FilterDenConstantOutMin=[]  FilterDenConstantOutMax=[]  PCopyOutDataTypeStr=Inherit: Inherit via back propagation  PCopyOutMin=[]  PCopyOutMax=[]  NCopyOutDataTypeStr=Inherit: Inherit via back propagation  NCopyOutMin=[]  NCopyOutMax=[]  IntegratorContinuousStateAttributes=''  IntegratorStateMustResolveToSignalObject=off  IntegratorRTWStateStorageClass=Auto  FilterContinuousStateAttributes=''  FilterStateMustResolveToSignalObject=off  FilterRTWStateStorageClass=Auto  ParallelPVariant=Passthrough  IdealPVariant=InternalParameters  IVariant=InternalParameters  DVariant=Disabled  IntegratorVariant=Continuous  SatVariant=Enabled  AWVariant=ContClampingIdeal  PCopyVariant=InternalParamsIdeal  TRVariant=Disabled  FdbkBlocksVariant=Forward  IdealPFdbkVariant=Disabled  SatFdbkVariant=Disabled  DerivativeFilterVariant=Disabled  NVariant=Disabled  NCopyVariant=Disabled_SignalSpec  FilterICVariant=Disabled  IntegratorICVariant=InternalICs  ExternalResetVariant=Disabled  TRSumVariant=Passthrough  SumFdbkVariant=Disabled  SumVariant=Sum_PI  TsampFilterVariant=InternalTs  TsampNgainVariant=Passthrough  TsampIntegralVariant=Disabled_SignalSpec  ExternalSaturationOutDataTypeStr=Inherit: Same as second input
  Product4 : Product
  S_initialize : $bdroot/general/S_initialize  SystemSampleTime=-1  VariantActivationTime=update diagram  AllowFlexibleInterface=on  Latency=0  AutoFrameSizeCalculation=off
  S_initialize1 : $bdroot/general/S_initialize  SystemSampleTime=-1  VariantActivationTime=update diagram  AllowFlexibleInterface=on  Latency=0  AutoFrameSizeCalculation=off
  Sum1 : Sum  Inputs=|+-
  Terminator : Terminator
  Terminator1 : Terminator
  Transfer Fcn (with initial states)1 : Subsystem  mask(Transfer Function with Initial States){N=[1], D=[300  1], X0=0}
      mask prompts: N "Numerator:"; D "Denominator:"; X0 "Initial conditions:"
      mask help: Vector expressions for numerator, and denominator. Coefficients are in descending powers of s.
      mask init:
      | [A,B,C,Dd]=tf2ss(N,D);if (isempty(X0));[m,n]=size(A);X0=zeros(1,m); end;
      mask Help: Specify the initial states for the transfer function.  The state ordering is determined by the m-file tf2ss.  There is no unique mapping of the states in a transfer function to states in a state-space representation.  However, tf2ss will consistently use the same mapping for a given transfer function.
      mask Display: dpoly(N,D,'s')
  convective : Gain  Gain=0.5  SaturateOnIntegerOverflow=on  OutDataTypeStr=Inherit: Same as input  ParamDataTypeStr=Inherit: Same as input
  heatload : Constant  Value=hvac.heatload
  radiative : Gain  Gain=0.5  SaturateOnIntegerOverflow=on  OutDataTypeStr=Inherit: Same as input  ParamDataTypeStr=Inherit: Same as input
  set point : Constant  Value=hvac.setpoint  VectorParams1D=off
  "[S1]" : Outport  InitialOutput=0  VectorParamsAs1DForOutWhenUnconnected=off
  "[S2]" : Outport  Port=2  InitialOutput=0  VectorParamsAs1DForOutWhenUnconnected=off
  "[HVACbus]" : Outport  Port=3  InitialOutput=0  VectorParamsAs1DForOutWhenUnconnected=off
  wires:
  Product4/1 -> Bus Assignment2/4, Bus Creator/1, Integrator/1, convective/1, radiative/1  "heating power"
  radiative/1 -> Bus Assignment2/2
  convective/1 -> Bus Assignment2/3
  heatload/1 -> Product4/2
  PID controller/1 -> Transfer Fcn (with initial states)1/1(In1)
  Bus Selector3/1 -> Sum1/1  "<Ts>"
  set point/1 -> Sum1/2
  Sum1/1 -> PID controller/1
  Bus Assignment2/1 -> "[S1]"/1
  WDB/1 -> Bus Selector1/1
  Transfer Fcn (with initial states)1/1(Out1) -> Product4/1
  AIB1/1 -> Bus Selector3/1
  Bus Selector1/1 -> Terminator/1  "<Temperature_Ambient>"
  S_initialize1/1 -> "[S2]"/1
  AIB2/1 -> Terminator1/1
  Bus Creator/1 -> "[HVACbus]"/1  "HVAC_999"
  Integrator/1 -> Bus Creator/2  "heating energy"
  S_initialize/1 -> Bus Assignment2/1

== system carnotUIBK_bus/airexchange_intersection/EMPTY ==
  AIB1 : Inport
  AIB2 : Inport  Port=2
  control : Inport  Port=3
  S_initialize : $bdroot/general/S_initialize  SystemSampleTime=-1  VariantActivationTime=update diagram  AllowFlexibleInterface=on  Latency=0  AutoFrameSizeCalculation=off
  S_initialize2 : $bdroot/general/S_initialize  SystemSampleTime=-1  VariantActivationTime=update diagram  AllowFlexibleInterface=on  Latency=0  AutoFrameSizeCalculation=off
  Selector1 : Selector  InputPortWidth=NUMBEROFCONTROLS  IndexOptions=Index vector (dialog)  Indices=[control]  OutputSizes=1
  Terminator : Terminator
  Terminator1 : Terminator
  Terminator2 : Terminator
  "[S1]" : Outport  InitialOutput=0  VectorParamsAs1DForOutWhenUnconnected=off
  "[S2]" : Outport  Port=2  InitialOutput=0  VectorParamsAs1DForOutWhenUnconnected=off
  wires:
  S_initialize/1 -> "[S1]"/1
  AIB2/1 -> Terminator2/1
  AIB1/1 -> Terminator1/1
  control/1 -> Selector1/1
  Selector1/1 -> Terminator/1
  S_initialize2/1 -> "[S2]"/1

== system carnotUIBK_bus/airexchange_intersection/airexchange_empiric ==
  note: ASSUMPTION: mdot_air_in = mdot_air_out !
  AIB1 : Inport
  AIB2 : Inport  Port=2
  control : Inport  Port=3
  1/3600 : Gain  Gain=1/3600
  Bus Assignment1 : BusAssignment  AssignedSignals=Qdotc,mdot_H2O,mdot_CO2,mdot_air,Qdot_V_infiltration
  Bus Assignment2 : BusAssignment  AssignedSignals=Qdotc,mdot_H2O,mdot_CO2,mdot_air,Qdot_T_neighbour
  Bus Selector1 : BusSelector  OutputSignals=Tc,x_H2O,x_CO2
  Bus Selector2 : BusSelector  OutputSignals=Tc,x_H2O,x_CO2,rho,cp
  Gain2 : Gain  Gain=0
  Gain3 : Gain  Gain=0
  Gain4 : Gain  Gain=-1
  Gain5 : Gain  Gain=-1
  Gain6 : Gain  Gain=-1
  Mux : Mux  Inputs=2
  Mux3 : Mux  Inputs=2
  Product2 : Product  InputSameDT=on  SaturateOnIntegerOverflow=on  OutDataTypeStr=Inherit: Same as first input
  Product4 : Product  Inputs=3  InputSameDT=on  SaturateOnIntegerOverflow=on  OutDataTypeStr=Inherit: Same as first input
  S_initialize : $bdroot/general/S_initialize  SystemSampleTime=-1  VariantActivationTime=update diagram  AllowFlexibleInterface=on  Latency=0  AutoFrameSizeCalculation=off
  S_initialize1 : $bdroot/general/S_initialize  SystemSampleTime=-1  VariantActivationTime=update diagram  AllowFlexibleInterface=on  Latency=0  AutoFrameSizeCalculation=off
  Selector1 : Selector  InputPortWidth=NUMBEROFCONTROLS  IndexOptions=Index vector (dialog)  Indices=[control]  OutputSizes=1
  Subsystem : Subsystem
  Sum : Sum  Inputs=-+  InputSameDT=on  SaturateOnIntegerOverflow=on  OutDataTypeStr=Inherit: Same as first input
  V exchange : Subsystem
  "[S1]" : Outport  InitialOutput=0  VectorParamsAs1DForOutWhenUnconnected=off
  "[S2]" : Outport  Port=2  InitialOutput=0  VectorParamsAs1DForOutWhenUnconnected=off
  wires:
  Sum/1 -> Product4/1  "dT"
  Bus Selector2/5 -> Product4/2  "<cp>"
  Bus Assignment2/1 -> "[S1]"/1
  Bus Selector2/3 -> Mux/2  "<x_CO2>"
  control/1 -> Selector1/1
  AIB1/1 -> Bus Selector2/1
  AIB2/1 -> Bus Selector1/1
  Bus Selector2/4 -> Product2/2  "<rho>"
  Product4/1 -> Bus Assignment2/6, Bus Assignment2/2, Gain4/1  "Qdot_air"
  Bus Selector2/2 -> V exchange/2(x in), Mux/1  "<x_H2O>"
  Mux/1 -> Subsystem/2(x_in)
  Mux3/1 -> Subsystem/3(x_out)
  Selector1/1 -> V exchange/5(control)
  Bus Assignment1/1 -> "[S2]"/1
  Bus Selector1/2 -> V exchange/4(x out), Mux3/1  "<x_H2O>"
  Bus Selector1/3 -> Mux3/2  "<x_CO2>"
  V exchange/1(V exchange) -> 1/3600/1
  Bus Selector1/1 -> Sum/2, V exchange/3(Tc out)  "<Tc>"
  Bus Selector2/1 -> Sum/1, V exchange/1(Tc in)  "<Tc>"
  1/3600/1 -> Product2/1
  Product2/1 -> Product4/3, Subsystem/1(mdot_air), Gain2/1, Gain3/1
  Gain3/1 -> Bus Assignment1/5
  Gain2/1 -> Bus Assignment2/5
  Subsystem/1(mdot_H2O) -> Gain5/1, Bus Assignment2/3  "mdot_H2O"
  S_initialize1/1 -> Bus Assignment1/1
  S_initialize/1 -> Bus Assignment2/1
  Gain4/1 -> Bus Assignment1/6, Bus Assignment1/2  "Qdot_air"
  Gain6/1 -> Bus Assignment1/4  "mdot_CO2"
  Subsystem/2(mdot_CO2) -> Gain6/1, Bus Assignment2/4  "mdot_CO2"
  Gain5/1 -> Bus Assignment1/3  "mdot_H2O"

== system carnotUIBK_bus/airexchange_intersection/airexchange_powerlaw ==
  note: ASSUMPTION: mdot_air_in = mdot_air_out !
  AIB1 : Inport
  AIB2 : Inport  Port=2
  control : Inport  Port=3
  Bus Assignment1 : BusAssignment  AssignedSignals=Qdotc,mdot_H2O,mdot_CO2,mdot_air,Qdot_T_neighbour
  Bus Assignment2 : BusAssignment  AssignedSignals=Qdotc,mdot_H2O,mdot_CO2,mdot_air,Qdot_T_neighbour
  Bus Selector2 : BusSelector  OutputSignals=Tc,x_H2O,x_CO2,rho
  Bus Selector3 : BusSelector  OutputSignals=Tc,x_H2O,x_CO2,rho,cp
  Constant18 : Constant  Value=zeros(1,9)
  Divide1 : Product  Inputs=*/
  Gain2 : Gain  Gain=0
  Gain3 : Gain  Gain=0
  Gain4 : Gain  Gain=-1
  Gain5 : Gain  Gain=-1
  Gain6 : Gain  Gain=-1
  Mux : Mux  Inputs=2
  Mux3 : Mux  Inputs=2
  Product4 : Product  Inputs=3  InputSameDT=on  SaturateOnIntegerOverflow=on  OutDataTypeStr=Inherit: Same as first input
  S_initialize : $bdroot/general/S_initialize  SystemSampleTime=-1  VariantActivationTime=update diagram  AllowFlexibleInterface=on  Latency=0  AutoFrameSizeCalculation=off
  S_initialize1 : $bdroot/general/S_initialize  SystemSampleTime=-1  VariantActivationTime=update diagram  AllowFlexibleInterface=on  Latency=0  AutoFrameSizeCalculation=off
  Selector1 : Selector  InputPortWidth=NUMBEROFCONTROLS  IndexOptions=Index vector (dialog)  Indices=[control]  OutputSizes=1
  Subsystem : Subsystem
  Sum : Sum  Inputs=-+  InputSameDT=on  SaturateOnIntegerOverflow=on  OutDataTypeStr=Inherit: Same as first input
  Transfer Fcn : TransferFcn  Denominator=[100 1]
  door open : Subsystem
  "door_area " : Constant  Value=area
  door_height : Constant  Value=height
  "door_height " : Constant  Value=height
  "[S1]" : Outport  InitialOutput=0  VectorParamsAs1DForOutWhenUnconnected=off
  "[S2]" : Outport  Port=2  InitialOutput=0  VectorParamsAs1DForOutWhenUnconnected=off
  wires:
  Sum/1 -> Product4/1  "dT"
  Bus Selector3/5 -> Product4/2  "<cp>"
  Bus Selector3/3 -> Mux/2  "<x_CO2>"
  control/1 -> Selector1/1
  AIB1/1 -> Bus Selector3/1
  AIB2/1 -> Bus Selector2/1
  Bus Selector2/1 -> Sum/2  "<Tc>"
  Bus Selector3/2 -> Mux/1  "<x_H2O>"
  Mux/1 -> Subsystem/2(x_in)
  Bus Selector3/1 -> Sum/1  "<Tc>"
  Mux3/1 -> Subsystem/3(x_out)
  Selector1/1 -> door open/5(control)
  door open/1(m_dot_open_door) -> Transfer Fcn/1
  Subsystem/2(mdot_CO2) -> Bus Assignment2/4, Gain4/1  "mdot_CO2"
  Subsystem/1(mdot_H2O) -> Gain5/1, Bus Assignment2/3  "mdot_H2O"
  Bus Selector2/2 -> Mux3/1  "<x_H2O>"
  Bus Selector2/3 -> Mux3/2  "<x_CO2>"
  door_height/1 -> door open/1(H (height of the door [m]))
  Divide1/1 -> door open/4(L)  "door width"
  Bus Selector3/4 -> door open/2(rho_i)  "<rho>"
  Bus Selector2/4 -> door open/3(rho_j)  "<rho>"
  "door_area "/1 -> Divide1/1
  "door_height "/1 -> Divide1/2
  Constant18/1 -> ?
  Gain3/1 -> Bus Assignment1/5
  Gain4/1 -> Bus Assignment1/4
  Gain5/1 -> Bus Assignment1/3
  Gain6/1 -> Bus Assignment1/2, Bus Assignment1/6
  Transfer Fcn/1 -> Gain3/1, Gain2/1, Subsystem/1(mdot_air), Product4/3
  S_initialize/1 -> Bus Assignment2/1
  Gain2/1 -> Bus Assignment2/5
  Product4/1 -> Bus Assignment2/6, Bus Assignment2/2, Gain6/1  "Qdot_air"
  Bus Assignment2/1 -> "[S1]"/1
  S_initialize1/1 -> Bus Assignment1/1
  Bus Assignment1/1 -> "[S2]"/1

== system carnotUIBK_bus/boundary/GDB ==
  GDB_create : BusCreator  Inputs=6
  ground_1 : FromWorkspace  VariableName=b.boundary.ground(1).temperature
  ground_2 : FromWorkspace  VariableName=b.boundary.ground(2).temperature
  ground_3 : FromWorkspace  VariableName=b.boundary.ground(3).temperature
  ground_4 : FromWorkspace  VariableName=b.boundary.ground(4).temperature
  ground_5 : FromWorkspace  VariableName=b.boundary.ground(5).temperature
  ground_6 : FromWorkspace  VariableName=b.boundary.ground(6).temperature
  GDB : Outport  VectorParamsAs1DForOutWhenUnconnected=off
  wires:
  ground_1/1 -> GDB_create/1  "ground_1"
  ground_3/1 -> GDB_create/3  "ground_3"
  ground_2/1 -> GDB_create/2  "ground_2"
  ground_6/1 -> GDB_create/6  "ground_6"
  ground_4/1 -> GDB_create/4  "ground_4"
  GDB_create/1 -> GDB/1
  ground_5/1 -> GDB_create/5  "ground_5"
